simulink model "SimpleVehicleModel"  (R2021b)
settings: Solver=VariableStepAuto  StartTime=0.0  StopTime=10.0  RelTol=1e-3
values from neighbouring files (symbols this model uses):
  AckermanFront = 0.2    [ForceBasedRollCenterModelWrapperScript.m]    (also in PlanarModelWrapperScriptAttempt2.m = 0; SimpleVehicleModelWrapperScript.m)
  AckermanRear = 0.1    [ForceBasedRollCenterModelWrapperScript.m]    (also in PlanarModelWrapperScriptAttempt2.m = 0; SimpleVehicleModelWrapperScript.m)
  Tire =     [3DOF Launch ControlHoosier_R25B_clean.mat]
  ToeFront = -0.0    (= 0)    [ForceBasedRollCenterModelWrapperScript.m]    (also in PlanarModelWrapperScriptAttempt2.m; SimpleVehicleModelWrapperScript.m)
  ToeRear = 0.0    (= 0)    [ForceBasedRollCenterModelWrapperScript.m]    (also in PlanarModelWrapperScriptAttempt2.m; SimpleVehicleModelWrapperScript.m)
settings Model: Creator=jpchi  LastModifiedBy=jpchi

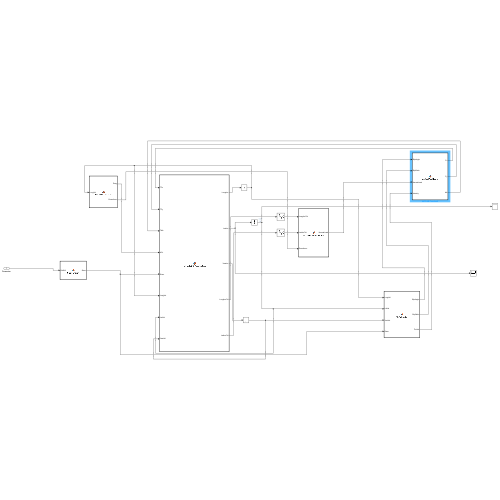
[thumbnail: Simulink's stored preview of the top-level diagram]
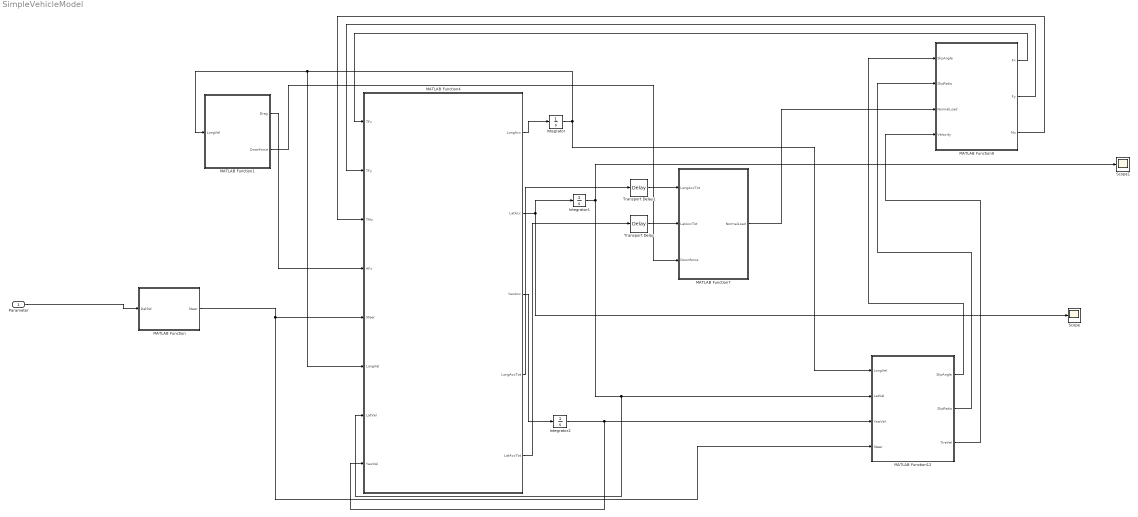
== system SimpleVehicleModel ==
  Parameter : Inport  OutMin=[-130]  OutMax=[130]  Unit=deg
  Integrator : Integrator
  Integrator1 : Integrator
  Integrator2 : Integrator
  MATLAB Function : MATLAB Function  TreatAsAtomicUnit=on
  MATLAB Function1 : MATLAB Function  TreatAsAtomicUnit=on
  MATLAB Function12 : MATLAB Function  TreatAsAtomicUnit=on
  MATLAB Function4 : MATLAB Function  TreatAsAtomicUnit=on
  MATLAB Function7 : MATLAB Function  TreatAsAtomicUnit=on
  MATLAB Function9 : MATLAB Function  TreatAsAtomicUnit=on
  Scope : Scope
  Scope1 : Scope
  Transport Delay : TransportDelay
  Transport Delay1 : TransportDelay
  wires:
  MATLAB Function9/1(Fx) -> MATLAB Function4/1(TFx)
  MATLAB Function12/3(TireVel) -> MATLAB Function9/4(Velocity)
  MATLAB Function12/2(SlipRatio) -> MATLAB Function9/2(SlipRatio)
  MATLAB Function12/1(SlipAngle) -> MATLAB Function9/1(SlipAngle)
  MATLAB Function9/2(Fy) -> MATLAB Function4/2(TFy)
  MATLAB Function7/1(NormalLoad) -> MATLAB Function9/3(NormalLoad)
  MATLAB Function4/1(LongAcc) -> Integrator/1
  MATLAB Function9/3(Mz) -> MATLAB Function4/3(TMz)
  MATLAB Function1/1(Drag) -> MATLAB Function4/4(AFx)
  MATLAB Function/1(Steer) -> MATLAB Function12/4(Steer), MATLAB Function4/5(Steer)
  MATLAB Function4/3(YawAcc) -> Integrator2/1
  MATLAB Function4/2(LatAcc) -> Integrator1/1, Scope/1
  MATLAB Function1/2(Downforce) -> MATLAB Function7/3(Downforce)
  Parameter/1 -> MATLAB Function/1(DelSW)
  Integrator2/1 -> MATLAB Function4/8(YawVel), MATLAB Function12/3(YawVel)
  Integrator/1 -> MATLAB Function12/1(LongVel), MATLAB Function4/6(LongVel), MATLAB Function1/1(LongVel)
  Integrator1/1 -> Scope1/1, MATLAB Function4/7(LatVel), MATLAB Function12/2(LatVel)
  MATLAB Function4/5(LatAccTot) -> Transport Delay/1
  MATLAB Function4/4(LongAccTot) -> Transport Delay1/1
  Transport Delay/1 -> MATLAB Function7/2(LatAccTot)
  Transport Delay1/1 -> MATLAB Function7/1(LongAccTot)

== matlab function SimpleVehicleModel/MATLAB Function1 ==
  data: LongVel input; Drag output size=1; Downforce output size=1; Parameter parameter
function [Drag, Downforce] = SimplifiedAeroLoads( LongVel, ...
    Parameter )
%% SimplifiedWeightTransfer - Simplified Normal Loads
% Computes tire normal loads using simplified weight transfer and
% aerodynamic loading.
% 
% Inputs:
%   LongVel    - (n,1 numeric) Longitudinal Velocity {dot{x}}  [m/s]
%   AirDensity - (n,1 numeric) Air Density           {rho_air} [kg/m^3]
%   RefArea    - (n,1 numeric) Reference Area        {A}       [m^2]
%   DragCoeff  - (n,1 numeric) Drag Coefficient      {C_D}     [ ]
%   LiftCoeff  - (n,1 numeric) Lift Coefficient      {C_L}     [ ]
%
% Outputs:
%   Drag       - (n,1 numeric) Drag Force            {A_F_x}   [N]
%   Downforce  - (n,1 numeric) Downforce             {A_F_z}   [N]
%
% Notes:
%
% Author(s): 
% Blake Christierson (bechristierson@ucdavis.edu) [Sep 2018 - Jun 2021] 
% 
% Last Updated: 31-May-2021

   
   

%% Computation
Drag      = 1/2 .* Parameter.AirDensity .*  Parameter.DragCoeff .* Parameter.RefArea .* LongVel.^2;
Downforce = 1/2 .* Parameter.AirDensity .* -Parameter.LiftCoeff .* Parameter.RefArea .* LongVel.^2;

end

== matlab function SimpleVehicleModel/MATLAB Function ==
  data: DelSW input; Steer output; ToeFront parameter; ToeRear parameter; AckermanFront parameter; AckermanRear parameter
function Steer      = SteerFunction( DelSW, ToeFront, ToeRear, AckermanFront, AckermanRear) 
%     Steer = @(DelSW, i) Parameter.Susp.Toe(1) .* (-1).^(mod(i,2)+1)        + ...
%         Parameter.Steer.MaxTire   .* (DelSW ./ Parameter.Steer.MaxWheel)     + ...
%         Parameter.Steer.Quadratic .* (DelSW ./ Parameter.Steer.MaxWheel).^2 .* (-1).^(mod(i,2)+1) + ...
%         Parameter.Steer.Cubic     .* (DelSW ./ Parameter.Steer.MaxWheel).^3  ;
Steer = [1:4]';
Steer(1) = -ToeFront + (DelSW + AckermanFront .* DelSW^2);
Steer(2) = ToeFront + (DelSW - AckermanFront .* DelSW^2);
Steer(3) = -ToeRear - (DelSW - AckermanRear .* DelSW^2);
Steer(4) = ToeRear - (DelSW + AckermanRear .* DelSW^2);


end

== matlab function SimpleVehicleModel/MATLAB Function4 ==
  data: TFx input; LongAcc output size=1; TFy input; TMz input; AFx input; Steer input; LongVel input; LatVel input; YawVel input; LatAcc output size=1; YawAcc output size=1; Parameter parameter; LongAccTot output; LatAccTot output
function [LongAcc, LatAcc, YawAcc, LongAccTot, LatAccTot] = ...
    FullTrack3DOFAccelerations( TFx, TFy, TMz, AFx, Steer, LongVel, LatVel, YawVel, Parameter)                                 
%% FullTrack3DOFAccelerations - Full Track Planar Accelerations
% Computes planar motion accelerations for a 3DOF full track chassis model
% 
% Inputs:
%   TFx        - (n,4 numeric) Tire Longitudinal Force {T_F_y}    [N]
%   TFy        - (n,4 numeric) Tire Lateral Force      {T_F_y}    [N]
%   TMz        - (n,4 numeric) Tire Aligning Moment    {T_M_z}    [N-m]
%   AFx        - (n,1 numeric) Aerodynamic Drag Force  {A_F_x}    [N]
%   AFy        - (n,1 numeric) Aerodynamic Side Force  {A_F_y}    [N]
%   AMz        - (n,1 numeric) Aerodynamic Yaw Moment  {A_M_z}    [N-m]
%   Wheelbase  - (n,1 numeric) Wheelbase               {L}        [m]
%   TrackWidth - (n,2 numeric) Track Width             {t_w}      [m]
%   Steer      - (n,4 numeric) Tire Steer Angle        {delta}    [deg]
%   Mass       - (n,1 numeric) Total Vehicle Mass      {m}        [kg]
%   YawInertia - (n,1 numeric) Vehicle Yaw Inertia     {I_zz}     [kg-m^2]
%   CoG        - (n,3 numeric) Center of Gravity       {CoG}      [m]
%   LongVel    - (n,1 numeric) Longitudinal Velocity   {dot{x}}   [m/s]
%   LatVel     - (n,1 numeric) Lateral Velocity        {dot{y}}   [m/s]
%   YawVel     - (n,1 numeric) Yaw Velocity            {dot{psi}} [rad/s]
%
% Outputs:
%   LongAcc    - (n,1 numeric) Longitudinal Acceleration       {ddot{x}}  [m/s^2]
%   LatAcc     - (n,1 numeric) Lateral Acceleration            {ddot{y}}  [m/s^2]
%   YawAcc     - (n,1 numeric) Yaw Acceleration                {ddot{psi} [rad/s^2]
%   LongAccTot - (n,1 numeric) Total Longitudinal Acceleration {a_x}      [m/s^2]
%   LatAccTot  - (n,1 numeric) Total Lateral Acceleration      {a_y}      [m/s^2]
%
% Notes:
%
% Author(s): 
% Blake Christierson (bechristierson@ucdavis.edu) [Sep 2018 - Jun 2021] 
% Tristan Pham       (atlpham@ucdavis.edu)        [Oct 2020 - ???     ]
% 
% Last Updated: 30-May-2021  

%% Computations
%%% Tire Positions (n,4,3 numeric)
TirePos = cat( 3, Parameter.Wheelbase/2 + [-1, -1, 1, 1].*Parameter.CoG(:,1), ...
                  [Parameter.TrackWidth(:,1).*[1 -1]/2, Parameter.TrackWidth(:,2).*[1 -1]/2], ...
                  zeros( size(Steer') ) );

%%% Tire Loads (n,4,3 numeric)
TireLoad = cat( 3, TFx, TFy, zeros( size(Steer') ) );

%%% Tire Yaw Moment (n,1 numeric)
TireMoment = cross(TirePos, TireLoad, 3);
TireMoment = sum( TireMoment(:,:,3) ) + sum(TMz,2);

%%% Chassis Accelerations
LongAcc = (sum( TFx.*cosd(Steer') - TFy.*sind(Steer'), 2 )  - AFx) ./ Parameter.Mass;  %Corriealus Term not included?+ LatVel.*YawVel
LatAcc  = (sum( TFy.*cosd(Steer') + TFx.*sind(Steer'), 2 )  - Parameter.AFy) ./ Parameter.Mass; %Corriealus Term Not Included?- LongVel.*YawVel
YawAcc  = (TireMoment - Parameter.AMz) ./ Parameter.YawInertia;

LongAccTot = LongAcc - LatVel .*YawVel;
LatAccTot  = LatAcc + LongVel .* YawVel;

== matlab function SimpleVehicleModel/MATLAB Function7 ==
  data: LongAccTot input; NormalLoad output size=[1 4]; LatAccTot input; Downforce input; Parameter parameter
function NormalLoad  = SimplifiedWeightTransfer( LongAccTot,...
         LatAccTot, Downforce, Parameter ) 
%% SimplifiedWeightTransfer - Simplified Normal Loads
% Computes tire normal loads using simplified weight transfer and
% aerodynamic loading.
% 
% Inputs:
%   LongAccTot - (n,1 numeric) Total Longitudinal Acceleration     {a_x}   [m/s^2]
%   LatAccTot  - (n,1 numeric) Total Lateral Acceleration          {a_y}   [m/s^2]
%   Wheelbase  - (n,1 numeric) Wheelbase                           {L}     [m]
%   TrackWidth - (n,2 numeric) Track Width                         {t_w}   [m]
%   Mass       - (n,1 numeric) Total Vehicle Mass                  {m}     [kg]
%   CoG        - (n,3 numeric) Center of Gravity                   {CoG}   [m]
%   Downforce  - (n,1 numeric) Aerodynamic Downforce               {A_F_z} [N]
%   CoP        - (n,3 numeric) Center of Pressure                  {CoP}   [m]
%   PerLLT     - (n,1 numeric) Percent Front Lateral Load Transfer {%_LLT} [ ]
%
% Outputs:
%   NormalLoad - (n,4 numeric) Tire Normal Loads                   {T_F_z} [N]
%
% Notes:
%
% Author(s): 
% Blake Christierson (bechristierson@ucdavis.edu) [Sep 2018 - Jun 2021] 
% 
% Last Updated: 30-May-2021
   
    
   

%% Computation
NormalLoad = zeros( [1, 4] );

%%% Total Weight Transfer
dFzx = Parameter.Mass .* LongAccTot .* Parameter.CoG(:,3) ./ Parameter.Wheelbase;
dFzy = Parameter.Mass .* LatAccTot  .* Parameter.CoG(:,3) ./ mean(Parameter.TrackWidth, 2);

%%% Static Wheel Loads
MassBal = (Parameter.CoG(:,1) + Parameter.Wheelbase./2) ./ Parameter.Wheelbase;
AeroBal = (Parameter.CoP(:,1) + Parameter.Wheelbase./2) ./ Parameter.Wheelbase;

NormalLoad(:,1:2) = (MassBal .* Parameter.Mass .* 9.81 + AeroBal .* Downforce) / 2;
NormalLoad(:,3:4) = ((1-MassBal) .* Parameter.Mass .* 9.81 + (1-AeroBal) .* Downforce) / 2;

%%% Dynamic Wheel Loads
NormalLoad(:,1) = NormalLoad(:,1) + (-0.5.*dFzx - Parameter.PerLLT    .*dFzy)/2;
NormalLoad(:,2) = NormalLoad(:,2) + (-0.5.*dFzx + Parameter.PerLLT    .*dFzy)/2;
NormalLoad(:,3) = NormalLoad(:,3) + ( 0.5.*dFzx - (1-Parameter.PerLLT).*dFzy)/2;
NormalLoad(:,4) = NormalLoad(:,4) + ( 0.5.*dFzx + (1-Parameter.PerLLT).*dFzy)/2;

end

== matlab function SimpleVehicleModel/MATLAB Function9 ==
  data: Fx output size=[1 4]; SlipAngle input; SlipRatio input; NormalLoad input; Velocity input; Fy output size=[1 4]; Mz output size=[1 4]; Parameter parameter; Tire parameter
function [Fx, Fy, Mz] = ContactPatchLoads( SlipAngle, SlipRatio, ...
    NormalLoad, Velocity, ...
    Parameter,  Tire) ...
%% ContactPatchLoads - Tire Load Evaluation
% This script evaluates a Pacejka contact patch tire model using the
% formatted by TireModelFittingMain(). 
% 
% Inputs:
%   Tire          - (struct)      Pacejka Parameters
%   SlipAngle     - (n,1 numeric) Slip Angle          {alpha} [deg]
%   SlipRatio     - (n,1 numeric) Slip Ratio          {kappa} [ ]
%   NormalLoad    - (n,1 numeric) Normal Load         {F_z}   [N]
%   Parameter.Pressure      - (n,1 numeric) Inflation Parameter.Pressure  {P_i}   [kPa]
%   Parameter.Inclination   - (n,1 numeric) Parameter.Inclination Angle   {gamma} [deg]
%   Velocity      - (n,1 numeric) Center Velocity     {v_c}   [m/s]
%   Parameter.Idx           - (n,1 numeric) Corner Parameter.Idx          {1-4}   [ ]
%   Model         - (struct)      Fidelity Choices 
%       .Pure     - (char)        Pure Slip Model     {'Linear', 'Pacejka'}
%       .Combined - (char)        Combined Slip Model {'Pure', 'MNC', 'Pacejka'}
%
% Outputs:
%   Fx - (n,1 numeric) Longitudinal (Tractive) Force {F_x} [N]
%   Fy - (n,1 numeric) Lateral Force                 {F_y} [N]
%   Mz - (n,1 numeric) Aligning Moment               {M_z} [N-m]
%   Mx - (n,1 numeric) Overturning Moment            {M_x} [N-m]
%   My - (n,1 numeric) Rolling Resistance            {M_y} [N-m]
%
% Notes:
%   Pacejka combined slip model is not currently implemented (4/2/21) and
%   when the model does become available the model compatibility checks
%   should be reformatted.
%
% Author(s): 
% Blake Christierson (bechristierson@ucdavis.edu) [Sep 2018 - Jun 2021] 
% Carlos Lopez       (calopez@ucdavis.edu       ) [Jan 2019 -         ]
% Leonardo Howard    (leohoward@ucdavis.edu     ) [Jan 2021 -         ]
% Tristan Pham       (atlpham@ucdavis.edu       ) [Jan 2021 -         ]
% 
% Last Updated: 23-Oct-2021
  

% %% Model Compatibility Check
% if ~ismember(Parameter.Model.Pure, {'Linear', 'Pacejka'})
%     error('Please choose either ''Linear'' or ''Pacejka'' for the pure slip model')
% elseif ~ismember(Parameter.Model.Combined, {'Pure', 'MNC'})
%     if strcmp(Parameter.Model.Combined, 'Pacejka')
%         error('The Pacejka combined slip model is not implemented (4/2/21)')
%     else
%         error('Please choose either ''Pure'' or ''MNC'' for the combined slip model')
%     end
% end

%% Main Evaluation
%%% Slip Angle Conversion
SlipAngle = deg2rad(SlipAngle);

%%% Left-Right Side Orientation Manipulation
% Ensures model conicity & ply-steer are symmetric to prevent drift
SlipAngle = SlipAngle .* (-1).^(mod(Parameter.Idx+1,2));
Parameter.Inclination   = Parameter.Inclination   .* (-1).^(mod(Parameter.Idx+1,2));

%%% Nondimensional Load & Parameter.Pressure
dFz = (NormalLoad - Tire.Pacejka.Fzo) ./ Tire.Pacejka.Fzo;
dPi = (Parameter.Pressure - Tire.Pacejka.Pio) ./ Tire.Pacejka.Pio;

%%% Evaluate Pure Slip Forces & Aligning Moment
[Fx0, Kxk, Kappa0] = EvaluateFx0( Tire, SlipAngle, SlipRatio, ...
    NormalLoad, dFz, Parameter.Pressure, dPi, Parameter.Inclination, Velocity, Parameter.Idx, Parameter.Model ); 

[Fy0, By, Cy, Kya, Hy, Vy, Alpha0] = EvaluateFy0( Tire, SlipAngle, SlipRatio, ...
    NormalLoad, dFz, Parameter.Pressure, dPi, Parameter.Inclination, Velocity, Parameter.Idx, Parameter.Model ); 
    
[Fyo, ~, ~, ~, ~, ~, Alphao] = EvaluateFy0( Tire, SlipAngle, SlipRatio, ...
    NormalLoad, dFz, Parameter.Pressure, dPi, 0  , Velocity, Parameter.Idx, Parameter.Model );

[Mz0, Bt, Ct, Dt, Et, Ht, Br, Cr, Dr, Hf] = EvaluateMz0( Tire, SlipAngle, SlipRatio, ...
    NormalLoad, dFz, Parameter.Pressure, dPi, Parameter.Inclination, Velocity, Parameter.Idx, Parameter.Model, ...
    Fyo, By, Cy, Kya, Hy, Vy );

%%% Combined Slip Force Models 
switch Parameter.Model.Combined
    case 'Pure' % Pure Slip Only Model
        Fx  = Fx0;
        Fy  = Fy0;   

    case 'MNC' % Modified-Nicolas-Comstock Combined Slip Model
        [Fx, Fy ]  = MNCCombinedSlipForces( Tire, ...
            SlipAngle, SlipRatio, Fx0, Fy0, Kxk, Kya, Kappa0, Alpha0 );
        [~ , Fyp]  = MNCCombinedSlipForces( Tire, ...
            SlipAngle, SlipRatio, Fx0, Fyo, Kxk, Kya, Kappa0, Alphao );

    case 'MF6_1' % Combined Slip Pacejka MF6.1 Model
        % Not Implemented
end

%%% Evaluate Combined Slip Aligning Moment (Mz)
if strcmpi( Parameter.Model.Combined, 'Pure' )
    Mz = Mz0;
else
    Mz = EvaluateMz( Tire, SlipAngle, SlipRatio, ...
        NormalLoad, dFz, Parameter.Pressure, dPi, Parameter.Inclination, Velocity, Parameter.Idx, Parameter.Model, ...
        Fx, Fy, Fyp, Kxk, Kya, Bt, Ct, Dt, Et, Ht, Br, Cr, Dr, Hf );
end

%%% Evaluate Moment & Rolling Resistance
% Mx = EvaluateMx( Tire, SlipAngle, SlipRatio, ...
%     NormalLoad, dFz, Parameter.Pressure, dPi, Parameter.Inclination, Velocity, Parameter.Idx, Model, Fy );
% 
% My = EvaluateMy( Tire, SlipAngle, SlipRatio, ...
%     NormalLoad, dFz, Parameter.Pressure, dPi, Parameter.Inclination, Velocity, Parameter.Idx, Model, Fx );

%%% Pure Slip Longitudinal Force Evaluation (Fx0)
function [Fx0, Kxk, Kappa0] = ...
        EvaluateFx0( Tire, ~, Kappa, Fz, dFz, ~, dPi, Inc, ~, ~, Model )
    Fx0 = [];
    Kxk = [];
    Kappa0 = [1 4];
    % Evaluate P6 Pacejka
    Cx = Tire.Pacejka.p.C.x(1) .* Tire.Pacejka.L.C.x;

    Dx = (Tire.Pacejka.p.D.x(1) + Tire.Pacejka.p.D.x(2).*dFz) .* ...
         (1 + Tire.Pacejka.p.P.x(3).*dPi + Tire.Pacejka.p.P.x(4).*dPi.^2) .* ...
         (1 - Tire.Pacejka.p.D.x(3).*Inc.^2).*Fz .* Tire.Pacejka.L.mu.x;

    Ex = ( Tire.Pacejka.p.E.x(1) + Tire.Pacejka.p.E.x(2).*dFz ...
        + Tire.Pacejka.p.E.x(3).*dFz.^2 ) .* ( 1 - Tire.Pacejka.p.E.x(4).*sign(Kappa) ) .* ...
        Tire.Pacejka.L.E.x;

    Kxk = Fz.*(Tire.Pacejka.p.K.x(1) + Tire.Pacejka.p.K.x(2).*dFz ) .* ...
        exp( Tire.Pacejka.p.K.x(3) .* dFz ) .* ...
        (1 + Tire.Pacejka.p.P.x(1).*dPi + Tire.Pacejka.p.P.x(2).*dPi.^2) .* ...
        Tire.Pacejka.L.K.x.k;

    Bx = Kxk ./ ( Cx.*Dx );

    Vx = Fz.*(Tire.Pacejka.p.V.x(1) + Tire.Pacejka.p.V.x(2).*dFz ) .* ...
        Tire.Pacejka.L.V.x;

    Hx = (Tire.Pacejka.p.H.x(1) + Tire.Pacejka.p.H.x(2).*dFz) .* ...
        Tire.Pacejka.L.H.x;

    % Evaluate Longitudinal Force​
    switch Model.Pure
        case 'Linear'
            Fx0 = Kxk .* Kappa;
        case 'Pacejka'
            Fx0 = Dx .* sin( Cx .* atan( (1-Ex) .* Bx.*(Kappa + Hx) + ...
                Ex.*atan( Bx.*(Kappa + Hx) ) ) ) + Vx;
    end

    % Evaluate Null Slip Ratio
    if strcmpi( Model.Combined, 'MNC' )
        Kappa0 = -Vx ./ Kxk - Hx;
        Kappa0(isnan(Kappa0)) = 0; % Can use smoothing in future
    else
        Kappa0 = [];
    end
 end

%%% Pure Slip Lateral Force Evaluation (Fy0)
function [Fy0, By, Cy, Kya, Hy, Vy, Alpha0] = ...
        EvaluateFy0( Tire, Alpha, ~, Fz, dFz, ~, dPi, Inc, ~, i, Model )            
   Alpha0 = [4 1];
   Fy0 = [];
   By = [];
   Cy = [];
   Kya = [];
   Hy = [];
   Vy = [];
    % Evaluate P6 Pacejka
    Cy = Tire.Pacejka.p.C.y(1);

    Dy = (Tire.Pacejka.p.D.y(1) + Tire.Pacejka.p.D.y(2).*dFz) .* ...
         (1 + Tire.Pacejka.p.P.y(3).*dPi + Tire.Pacejka.p.P.y(4).*dPi.^2) .* ...
         (1 - Tire.Pacejka.p.D.y(3).*Inc.^2).*Fz;

    Kya = Tire.Pacejka.p.K.y(1) .* Tire.Pacejka.Fzo .* ( 1 + Tire.Pacejka.p.P.y(1).*dPi ) .* ...
        ( 1 - Tire.Pacejka.p.K.y(3).*abs(Inc) ) .* sin( Tire.Pacejka.p.K.y(4) .* ...
        atan( (Fz./Tire.Pacejka.Fzo) ./ ...
        ( ( Tire.Pacejka.p.K.y(2) + Tire.Pacejka.p.K.y(5).*Inc.^2 ) .* ...
        ( 1 + Tire.Pacejka.p.P.y(2).*dPi ) ) ) );

    Kyg0 = Fz.*(Tire.Pacejka.p.K.y(6) + Tire.Pacejka.p.K.y(7).*dFz ) .* ...
        (1 + Tire.Pacejka.p.P.y(5).*dPi );

    By = Kya ./ ( Cy.*Dy );

    Vyg = Fz.*(Tire.Pacejka.p.V.y(3) + Tire.Pacejka.p.V.y(4).*dFz ).*Inc;

    Vy = Fz.*(Tire.Pacejka.p.V.y(1) + Tire.Pacejka.p.V.y(2).*dFz ) + Vyg;

    Hy = (Tire.Pacejka.p.H.y(1) + Tire.Pacejka.p.H.y(2).*dFz ) .* (Kyg0.*Inc - Vyg ) ./ Kya;

    Ey = ( Tire.Pacejka.p.E.y(1) + Tire.Pacejka.p.E.y(2).*dFz ) .* ...
        ( 1 + Tire.Pacejka.p.E.y(5).*Inc.^2 - ...
        ( Tire.Pacejka.p.E.y(3) + Tire.Pacejka.p.E.y(4).*Inc ).*sign(Alpha + Hy) );

    % Evaluate Lateral Force
    switch Model.Pure
        case 'Linear'
            Fy0 = Kya .* Alpha;
        case 'Pacejka'
            Fy0 = (Dy .* sin( Cy .* atan( (1-Ey) .* By.*( Alpha + Hy ) + ...
                Ey .* atan( By.*( Alpha + Hy ) ) ) ) + Vy) .* (-1).^(mod(i+1,2));
    end

    % Evaluate Null Slip Angle
    if strcmpi( Model.Combined, 'MNC' )
        Alpha0 = -Vy ./ Kya - Hy;
        Alpha0(isnan(Alpha0)) = 0;
    else
        Alpha0 = [];
    end
end

%%% Evaluate Pure Slip Aligning Moment (Mz0)
function [Mz0, Bt, Ct, Dt, Et, Ht, Br, Cr, Dr, Hf] = ...
        EvaluateMz0( Tire, Alpha, ~, Fz, dFz, ~, dPi, Inc, ~, i, ~, ...
            Fyo, By, Cy, Kya, Hy, Vy )
    
    % Evaluate P6 Pacejka
    Bt = (Tire.Pacejka.q.B.z(1) + Tire.Pacejka.q.B.z(2).*dFz + ...
        Tire.Pacejka.q.B.z(3).*dFz.^2) .* ...
        (1 + Tire.Pacejka.q.B.z(5).*abs(Inc) + ...
        Tire.Pacejka.q.B.z(6).*Inc.^2);

    Ct = Tire.Pacejka.q.C.z(1);

    Dt = (Tire.Pacejka.Ro ./ Tire.Pacejka.Fzo) .* ...
        ( Tire.Pacejka.q.D.z(5) .* (Tire.Pacejka.Fzo ./ Tire.Pacejka.Ro) + ...
        Tire.Pacejka.q.D.z(1).*Fz + Tire.Pacejka.q.D.z(2).*Fz.*dFz ) .* ...
        ( 1 - Tire.Pacejka.p.P.z(1).*dPi ) .* ...
        ( 1 + Tire.Pacejka.q.D.z(3).*abs(Inc) + ...
        Tire.Pacejka.q.D.z(4).*Inc.^2 );

    Ht = Tire.Pacejka.q.H.z(1) + ...
        Tire.Pacejka.q.H.z(2).*dFz + (Tire.Pacejka.q.H.z(3) + ...
        Tire.Pacejka.q.H.z(4).*dFz).*Inc;

    Et = (Tire.Pacejka.q.E.z(1) + Tire.Pacejka.q.E.z(2).*dFz + ...
        Tire.Pacejka.q.E.z(3).*dFz.^2) .* ...
        (1 + (Tire.Pacejka.q.E.z(4) + Tire.Pacejka.q.E.z(5).*Inc).*(2/pi).* ...
        atan( Bt .* Ct .* (Alpha+Ht) ) );

    Br = Tire.Pacejka.q.B.z(10) .* By .* Cy;

    Cr = 1;

    Dr = Tire.Pacejka.Ro .* Fz .* ( ( Tire.Pacejka.q.D.z(6) + ...
        Tire.Pacejka.q.D.z(7).*dFz ) + ...
        ( ( Tire.Pacejka.q.D.z(8) + Tire.Pacejka.q.D.z(9).*dFz ) .* ...
        ( 1 + Tire.Pacejka.p.P.z(2).*dPi ) + ...
        ( Tire.Pacejka.q.D.z(10) + Tire.Pacejka.q.D.z(11).*dFz ) .* ...
        abs(Inc) ).*Inc ) .* cos( Alpha );

    Hf = Hy + Vy ./ Kya;

    % Evaluate Trail Function
    t0 = Dt.*cos( Ct.*atan( (1-Et).*(Bt.*(Alpha + Ht)) + ...
        Et.*atan( Bt.*(Alpha + Ht) ) ) ) .* cos( Alpha ) ;

    % Evaluate Residual Aligning Moment
    Mzro = Dr .* cos( Cr.*atan( Br.*(Alpha + Hf) ) ).* cos( Alpha );

    % Evaluate Pure Slip Aligning Moment (Mz0)
    Mz0 = (-t0 .* Fyo .* (-1).^(mod(i+1,2)) + Mzro) .* (-1).^(mod(i+1,2));
end

%%% Modified-Nicolas Comstock Combined Slip Forces
function [Fx, Fy] = MNCCombinedSlipForces( ~, Alpha, Kappa, Fx0, Fy0, Kxk, Kya, Kappa0, Alpha0 )
    Fx = abs(Fx0 .* Fy0 ./ sqrt( (Kappa - Kappa0).^2 .* Fy0.^2 + Fx0.^2 .* tan(Alpha - Alpha0).^2 ) .* ...
        sqrt( (Kappa - Kappa0).^2 .* Kya.^2 + (1 - abs(Kappa - Kappa0)).^2 .* cos(Alpha - Alpha0).^2 .* Fx0.^2 ) ./ Kya) .* sign(Fx0);

    Fy = abs( Fx0 .* Fy0 ./ sqrt( (Kappa - Kappa0).^2 .* Fy0.^2 + Fx0.^2 .* tan(Alpha - Alpha0).^2 ) .* ...
        sqrt( (1 - abs(Kappa - Kappa0)).^2 .* cos(Alpha - Alpha0).^2 .* Fy0.^2 + sin(Alpha - Alpha0).^2 .* Kxk.^2 ) ./ ...
        ( Kxk .* cos(Alpha - Alpha0)) ) .* sign(Fy0);
end

%%% Evaluate Combined Slip Aligning Moment (Mz)
function Mz = EvaluateMz( Tire, Alpha, Kappa, ~, dFz, ~, ~, Inc, ~, i, ~, ...
    Fx, Fy, Fyp, Kxk, Kya, Bt, Ct, Dt, Et, Ht, Br, Cr, Dr, Hf )
    
    % Equivalent Slips
    Alphat = (Alpha + (-1).^(mod(i+1,2)).*Ht );
    Alphar = (Alpha + (-1).^(mod(i+1,2)).*Hf );

    Alphateq = sqrt( Alphat.^2 + (Kxk./Kya).^2 .* Kappa.^2 ) .* sign( Alphat );
    Alphareq = sqrt( Alphar.^2 + (Kxk./Kya).^2 .* Kappa.^2 ) .* sign( Alphar );

    % Evaluate Trail Function
    t = Dt.*cos( Ct.*atan( (1-Et).*(Bt.*Alphateq) + ...
        Et.*atan(Bt.*Alphateq) ) ) .* cos( Alpha );

    % Evaluate Scrub Function
    s = Tire.Pacejka.Ro .* (Tire.Pacejka.s.s.z(1) + ...
        Tire.Pacejka.s.s.z(2) .* (Fy./Tire.Pacejka.Fzo) + ...
        (Tire.Pacejka.s.s.z(3) + Tire.Pacejka.s.s.z(4) .* dFz) .* Inc );

    % Evaluate Residual Aligning Moment
    Mzr = Dr .* cos( Cr.*atan( Br.*(Alphareq) ) ) .* cos( Alpha );

    % Evaluate Pure Slip Aligning Moment (Mz0)
    Mz = -t .* Fyp + Mzr + s .* Fx;
end

%%% Evaluate Overturning Moment
% function Mx = EvaluateMx( Tire, ~, ~, Fz, ~, ~, dPi, Inc, ~, ~, ~, Fy )
%     Mx = Tire.Pacejka.Ro .* Fz .* ( Tire.Pacejka.q.s.x(1) - ...
%         Tire.Pacejka.q.s.x(2) .* Inc .* ( 1 + Tire.Pacejka.p.P.Mx(1).*dPi ) + ...
%         Tire.Pacejka.q.s.x(3) .* Fy ./ Tire.Pacejka.Fzo + ...
%         Tire.Pacejka.q.s.x(4) .* cos( Tire.Pacejka.q.s.x(5) .* ...
%         ( atan( (Tire.Pacejka.q.s.x(6) .* Fz ./ Tire.Pacejka.Fzo) ) ).^2 ) .* ...
%         sin( Tire.Pacejka.q.s.x(7) .* Inc + Tire.Pacejka.q.s.x(8) .* ...
%         atan( Tire.Pacejka.q.s.x(9) .* Fy ./ Tire.Pacejka.Fzo ) ) + ...
%         Tire.Pacejka.q.s.x(10) .* atan( Tire.Pacejka.q.s.x(11) .* Fz ./ Tire.Pacejka.Fzo ) .* Inc );
% end
% 
% %%% Evaluate Rolling Resistance
% function My = EvaluateMy( Tire, ~, Kappa, Fz, ~, Pi, ~, ~, V, ~, ~, Fx )
%     Re = Tire.Radius.Effective( Kappa, Fz, Pi );
%     Rl = Tire.Radius.Loaded( Fz, Pi );
%     
%     My = Fx .* (Re - Rl) + Fz .* Re .* ( Tire.Pacejka.q.s.y(1) + ...
%         Tire.Pacejka.q.s.y(3) .* (V ./ Tire.Pacejka.Vo) + ...
%         Tire.Pacejka.q.s.y(4) .* (V ./ Tire.Pacejka.Vo).^4 );
% end

end

== matlab function SimpleVehicleModel/MATLAB Function12 ==
  data: LongVel input; SlipAngle output size=[1 4]; LatVel input; YawVel input; Steer input; SlipRatio output size=[1 4]; TireVel output size=[4 3]; Parameter parameter
function [SlipAngle, SlipRatio, TireVel] = SlipEstimation( ...
    LongVel, LatVel, YawVel, Steer, Parameter)

%% SlipEstimation - Slip Angle and Slip Ratio Calculations
% Estimates tire slips and center velocity from chassis velocity and a
% handful of tire states.
% 
% Inputs:
%   LongVel   - (1,1 numeric) Longitudinal Velocity {x_dot}   [m/s]
%   LatVel    - (1,1 numeric) Lateral Velocity      {y_dot}   [m/s]
%   YawVel    - (1,1 numeric) Yaw Rate              {psi_dot} [rad/s]
%   TirePos   - (n,3 numeric) [x,y,0] Tire Position {p}       [m]
%   Steer     - (n,1 numeric) Tire Steer Angle      {delta}   [deg]
%   SpinRate  - (n,1 numeric) Tire Spin Rate        {omega}   [rad/s]
%   EffRadius - (n,1 numeric) Tire Effective Radius {r_e}     [m]
% 
% Outputs:
%   SlipAngle - (n,1 numeric) Tire Slip Angle      {alpha} [deg]
%   SlipRatio - (n,1 numeric) Tire Slip Ratio      {kappa} [ ]
%   TireVel   - (n,1 numeric) Tire Center Velocity {v_c}   [m/s]
%
% Notes:
%   Typically n=4; however, may be vectorized by stacking rows.
%
% Author(s): 
% Blake Christierson (bechristierson@ucdavis.edu) [Sep 2018 - Jun 2021] 
%
% Last Updated: 1-Apr-2021

   
%% Computation
%%% Number of Evaluations
n = numel(Steer);

%%% Tire Center Velocities
TireVel = zeros(n,3);
for i = 1:n
    TireVel(i,:) = [LongVel; LatVel; 0] + cross( [0; 0; YawVel], Parameter.TirePos(i,:)' );
end

%%% Slip Angle
SlipAngles = atan2d( TireVel(:,2), TireVel(:,1) ) - Steer;
SlipAngle = SlipAngles';

%%% Slip Ratio
SlipRatios = ( Parameter.SpinRate .* Parameter.EffRadius ) ./ ( norm(TireVel,2) .* cosd( SlipAngle' ) ) - 1;
SlipRatio = SlipRatios';
